simulink model "UseSimSensorData"  (R2018b)
settings: configuration reference "RPi_DynamicsRate" (kept outside this file)
values from neighbouring files (symbols this model uses):
  M_IMU_To_Body = euler2mat(Euler_IMU_To_Body)    [loadSensorData.m]
undefined symbols (not defined in the file or in its folder): DiscIntNeverNeededParam
settings Model: Creator=barthal  LastModifiedBy=barthal
settings ConfigSetRef: SourceLocation=Base Workspace

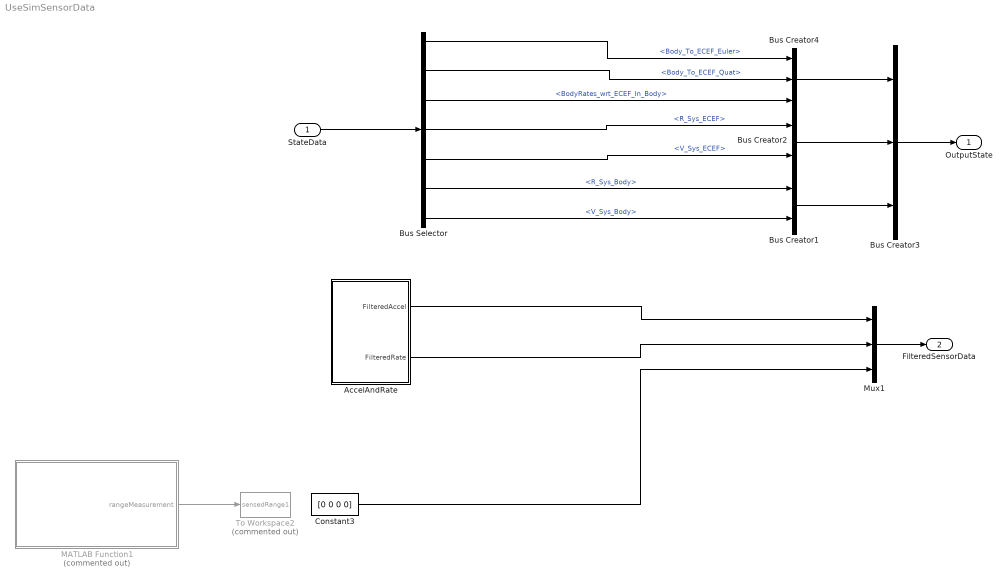
== system UseSimSensorData ==
  StateData : Inport  OutDataTypeStr=Bus: FullStateBus
  AccelAndRate : Subsystem
  Bus Creator1 : BusCreator  Inputs=2  OutDataTypeStr=Bus: TranStateBodyBus
      settings: InheritFromInputs=off
  Bus Creator2 : BusCreator  Inputs=2  OutDataTypeStr=Bus: TranStateECEFBus
      settings: InheritFromInputs=off
  Bus Creator3 : BusCreator  Inputs=3  OutDataTypeStr=Bus: FullStateBus
      settings: InheritFromInputs=off
  Bus Creator4 : BusCreator  Inputs=3  OutDataTypeStr=Bus: RotStateBodyECEFBus
      settings: InheritFromInputs=off
  Bus Selector : BusSelector  OutputSignals=RotState_Body_ECEF.Body_To_ECEF_Euler,RotState_Body_ECEF.Body_To_ECEF_Quat,RotState_Body_ECEF.BodyRates_wrt_ECEF_In_Body,TranState_ECEF.R_Sys_ECEF,TranState_ECEF.V_Sys_ECEF,TranState_Body.R_Sys_Body,TranState_Body.V_Sys_Body
  Constant3 : Constant  Value=[0 0 0 0]
  MATLAB Function1 : MATLAB Function  Commented=on  TreatAsAtomicUnit=on
  Mux1 : Mux  Inputs=3
  To Workspace2 : ToWorkspace  Commented=on  VariableName=sensedRange1  SaveFormat=Timeseries  SampleTime=-1
  OutputState : Outport  OutDataTypeStr=Bus: FullStateBus
  FilteredSensorData : Outport  Port=2
  wires:
  AccelAndRate/2(FilteredRate) -> Mux1/2
  AccelAndRate/1(FilteredAccel) -> Mux1/1
  Constant3/1 -> Mux1/3
  Mux1/1 -> FilteredSensorData/1
  Bus Selector/3 -> Bus Creator4/3  "<BodyRates_wrt_ECEF_In_Body>"
  Bus Selector/2 -> Bus Creator4/2  "<Body_To_ECEF_Quat>"
  Bus Selector/5 -> Bus Creator2/2  "<V_Sys_ECEF>"
  Bus Creator2/1 -> Bus Creator3/2
  Bus Creator1/1 -> Bus Creator3/3
  Bus Selector/7 -> Bus Creator1/2  "<V_Sys_Body>"
  MATLAB Function1/1(rangeMeasurement) -> To Workspace2/1
  Bus Creator4/1 -> Bus Creator3/1
  Bus Selector/4 -> Bus Creator2/1  "<R_Sys_ECEF>"
  StateData/1 -> Bus Selector/1
  Bus Selector/1 -> Bus Creator4/1  "<Body_To_ECEF_Euler>"
  Bus Creator3/1 -> OutputState/1
  Bus Selector/6 -> Bus Creator1/1  "<R_Sys_Body>"

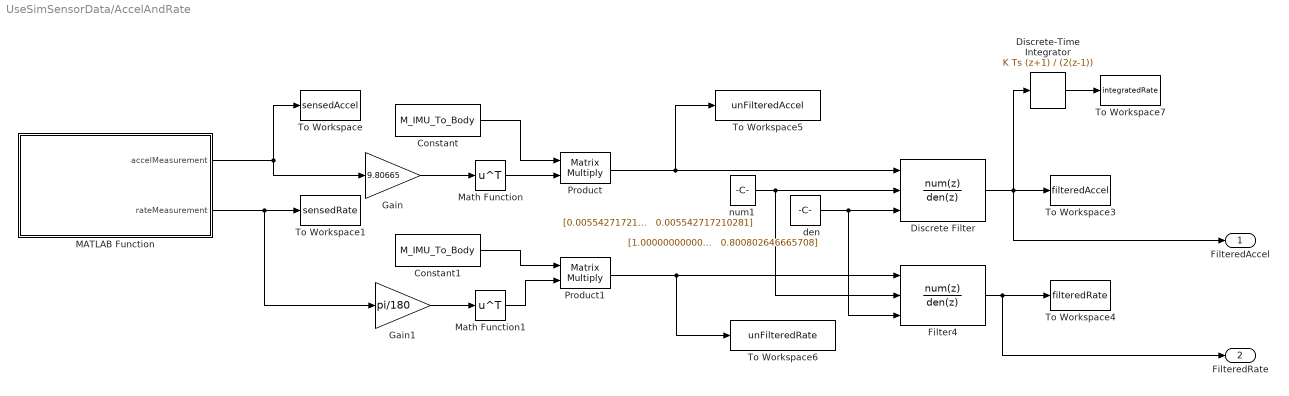
== system UseSimSensorData/AccelAndRate ==
  Constant : Constant  Value=M_IMU_To_Body
  Constant1 : Constant  Value=M_IMU_To_Body
  Discrete Filter : DiscreteFilter  NumeratorSource=Input port  DenominatorSource=Input port  a0EqualsOne=on
      settings: InputPortMap=u0,p1,p3
  Discrete-Time Integrator : DiscreteIntegrator  IntegratorMethod=Integration: Trapezoidal  SampleTime=-1  ICPrevOutput=DiscIntNeverNeededParam  ICPrevScaledInput=DiscIntNeverNeededParam
  Filter4 : DiscreteFilter  Tag=BlockMethodSubSystem  NumeratorSource=Input port  Numerator=[2.46193004641406277e-06 4.92386009282812554e-06 2.46193004641406277e-06]  DenominatorSource=Input port  Denominator=[1 -1.99555712434578902 0.995566972065974776]  a0EqualsOne=on
      settings: InputPortMap=u0,p1,p3
  Gain : Gain  Gain=9.80665
  Gain1 : Gain  Gain=pi/180
  MATLAB Function : MATLAB Function  TreatAsAtomicUnit=on
  Math Function : Math  Operator=transpose  SaturateOnIntegerOverflow=on
  Math Function1 : Math  Operator=transpose  SaturateOnIntegerOverflow=on
  Product : Product  Multiplication=Matrix(*)
  Product1 : Product  Multiplication=Matrix(*)
  To Workspace : ToWorkspace  VariableName=sensedAccel  SaveFormat=Timeseries  SampleTime=-1
  To Workspace1 : ToWorkspace  VariableName=sensedRate  SaveFormat=Timeseries  SampleTime=-1
  To Workspace3 : ToWorkspace  VariableName=filteredAccel  SaveFormat=Timeseries  SampleTime=-1
  To Workspace4 : ToWorkspace  VariableName=filteredRate  SaveFormat=Timeseries  SampleTime=-1
  To Workspace5 : ToWorkspace  VariableName=unFilteredAccel  SaveFormat=Timeseries  SampleTime=-1
  To Workspace6 : ToWorkspace  VariableName=unFilteredRate  SaveFormat=Timeseries  SampleTime=-1
  To Workspace7 : ToWorkspace  VariableName=integratedRate  SaveFormat=Timeseries  SampleTime=-1
  den : Constant  Value="[1.000000000000000  -1.778631777824585   0.800802646665708]"
  num1 : Constant  Value="[0.005542717210281   0.011085434420561   0.005542717210281]"  VectorParams1D=off
  FilteredAccel : Outport
  FilteredRate : Outport  Port=2
  wires:
  Product/1 -> To Workspace5/1, Discrete Filter/1
  Discrete Filter/1 -> FilteredAccel/1, Discrete-Time Integrator/1, To Workspace3/1
  Product1/1 -> To Workspace6/1, Filter4/1
  Filter4/1 -> FilteredRate/1, To Workspace4/1
  num1/1 -> Filter4/2, Discrete Filter/2
  MATLAB Function/2(rateMeasurement) -> Gain1/1, To Workspace1/1
  den/1 -> Filter4/3, Discrete Filter/3
  MATLAB Function/1(accelMeasurement) -> To Workspace/1, Gain/1
  Discrete-Time Integrator/1 -> To Workspace7/1
  Gain/1 -> Math Function/1
  Constant/1 -> Product/1
  Constant1/1 -> Product1/1
  Gain1/1 -> Math Function1/1
  Math Function/1 -> Product/2
  Math Function1/1 -> Product1/2

== matlab function UseSimSensorData/AccelAndRate/MATLAB Function ==
  data: accelMeasurement output; rateMeasurement output
function [accelMeasurement,rateMeasurement]= callgetAccelPhidgetData()

% These variables must be persistent to ensure the attachment to the
% sensor channel is maintained
persistent accelPhidget gyroPhidget 

% Not all python functions seem to be able to be called from a Matlab 
% function block, so the entire function is considered extrinsic
coder.extrinsic('getAccelPhidgetData');
coder.extrinsic('py.Accelerometer.Accelerometer');
coder.extrinsic('py.Gyroscope.Gyroscope');

% Create the channel to the sensor
% This code needs error handling
if isempty(accelPhidget)
    accelPhidget = py.Accelerometer.Accelerometer;
end
if isempty(gyroPhidget)
    gyroPhidget = py.Gyroscope.Gyroscope;
end

% The data types need to be pre-allocated
accelMeasurement = [0 0 0];
rateMeasurement = [0 0 0];
accelTimestamp = 0;
rateTimestamp = 0;

% Get the sensor data
[accelMeasurement,rateMeasurement,accelTimestamp,rateTimestamp] = getAccelPhidgetData(accelPhidget,gyroPhidget);

== matlab function UseSimSensorData/MATLAB Function1 ==
  data: rangeMeasurement output
function rangeMeasurement  = callgetRangePhidgetData()

% These variables must be persistent to ensure the attachment to the
% sensor channel is maintained
persistent rangePhidget1 rangePhidget2 rangePhidget3 rangePhidget4

% Not all python functions seem to be able to be called from a Matlab 
% function block, so the entire function is considered extrinsic
coder.extrinsic('getRangePhidgetData');
coder.extrinsic('py.DistanceSensor.DistanceSensor');

% Create the channel to the sensor
% This code needs error handling
if isempty(rangePhidget1)
    rangePhidget1 = py.DistanceSensor.DistanceSensor;
end
if isempty(rangePhidget2)
    rangePhidget2 = py.DistanceSensor.DistanceSensor;
end
if isempty(rangePhidget3)
    rangePhidget3 = py.DistanceSensor.DistanceSensor;
end
if isempty(rangePhidget4)
    rangePhidget4 = py.DistanceSensor.DistanceSensor;
end

% The data types need to be pre-allocated
rangeMeasurement = [0 0 0 0];

% Get the sensor data
[rangeMeasurement] = getRangePhidgetData(rangePhidget1,rangePhidget2,rangePhidget3,rangePhidget4);
